simulink model "DREM"  (R2022a)
settings: Solver=FixedStepAuto  StartTime=0.0  StopTime=50.0  FixedStep=0.001  RelTol=1e-6
libraries: cstblocks x3
settings Model: Creator=loryb  LastModifiedBy=loryb

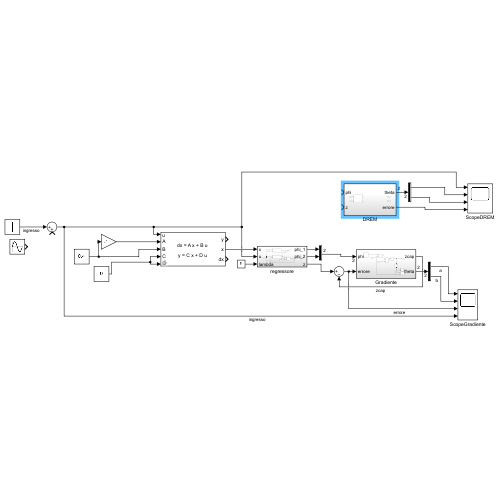
[thumbnail: Simulink's stored preview of the top-level diagram]
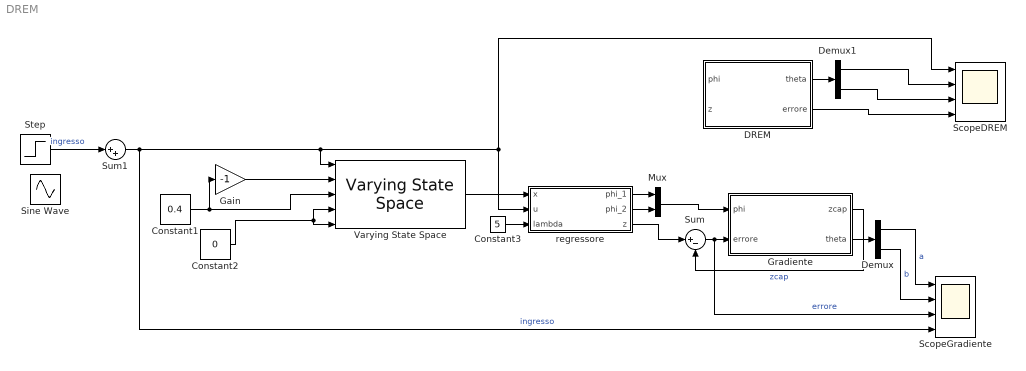
== system DREM ==
  Constant1 : Constant  Value=0.4
  Constant2 : Constant  Value=0
  Constant3 : Constant  Value=5
  DREM : Subsystem
  Demux : Demux  Outputs=2
  Demux1 : Demux  Outputs=2
  Gain : Gain  Gain=-1
  Gradiente : Subsystem
  Mux : Mux  Inputs=2
  ScopeDREM : Scope  NumInputPorts=4
  ScopeGradiente : Scope  NumInputPorts=4
  Sine Wave : Sin  Amplitude=10  Frequency=5/2  SampleTime=0
  Step : Step  Time=3  After=10  SampleTime=0
  Sum : Sum  Inputs=|+-
  Sum1 : Sum  Inputs=|++
  Varying State Space : cstblocks/Linear Parameter Varying/Varying State Space  x0=0  xNames=''  OutputX=on  OutputDX=on
  regressore : Subsystem
  wires:
  Gain/1 -> Varying State Space/2
  Constant1/1 -> Gain/1, Varying State Space/3
  Constant2/1 -> Varying State Space/4, Varying State Space/5
  Varying State Space/2 -> regressore/1(x)
  Constant3/1 -> regressore/3(lambda)
  Sum/1 -> ScopeGradiente/3, Gradiente/2(errore)  "errore"
  Gradiente/1(zcap) -> Sum/2  "zcap"
  regressore/3(z) -> Sum/1
  Sum1/1 -> Varying State Space/1, ScopeDREM/1, regressore/2(u), ScopeGradiente/4  "ingresso"
  Demux/2 -> ScopeGradiente/2  "b"
  Demux/1 -> ScopeGradiente/1  "a"
  regressore/2(phi_2) -> Mux/2
  regressore/1(phi_1) -> Mux/1
  Mux/1 -> Gradiente/1(phi)
  Gradiente/2(theta) -> Demux/1
  Step/1 -> Sum1/1  "ingresso"
  DREM/2(errore) -> ScopeDREM/4
  DREM/1(theta) -> Demux1/1
  Demux1/1 -> ScopeDREM/2
  Demux1/2 -> ScopeDREM/3

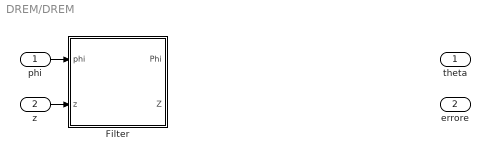
== system DREM/DREM ==
  phi : Inport
  z : Inport  Port=2
  Filter : Subsystem
  theta : Outport
  errore : Outport  Port=2
  wires:
  z/1 -> Filter/2(z)
  phi/1 -> Filter/1(phi)

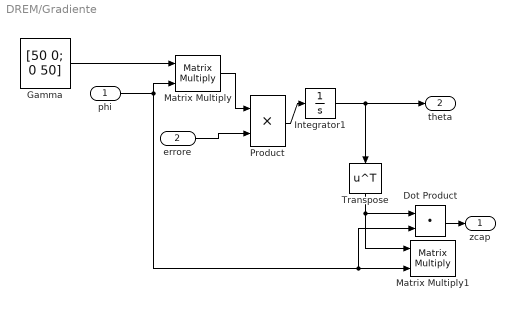
== system DREM/Gradiente ==
  phi : Inport
  errore : Inport  Port=2
  Dot Product : DotProduct  OutDataTypeStr=Inherit: Inherit via internal rule
  Gamma : Constant  Value=[50 0; 0 50]  VectorParams1D=off
  Integrator1 : Integrator
  Matrix Multiply : Product  Multiplication=Matrix(*)
  Matrix Multiply1 : Product  Multiplication=Matrix(*)
  Product : Product
  Transpose : Math  Operator=transpose
  zcap : Outport
  theta : Outport  Port=2
  wires:
  Gamma/1 -> Matrix Multiply/1
  phi/1 -> Matrix Multiply/2, Dot Product/2, Matrix Multiply1/2
  Product/1 -> Integrator1/1
  errore/1 -> Product/2
  Matrix Multiply/1 -> Product/1
  Integrator1/1 -> Transpose/1, theta/1
  Transpose/1 -> Matrix Multiply1/1, Dot Product/1
  Dot Product/1 -> zcap/1

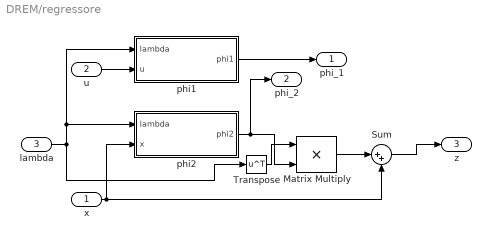
== system DREM/regressore ==
  x : Inport
  u : Inport  Port=2
  lambda : Inport  Port=3
  Matrix Multiply : Product
  Sum : Sum  Inputs=|++
  Transpose : Math  Operator=transpose
  phi1 : Subsystem
  phi2 : Subsystem
  phi_1 : Outport
  phi_2 : Outport  Port=2
  z : Outport  Port=3
  wires:
  x/1 -> Sum/2, phi2/2(x)
  u/1 -> phi1/2(u)
  lambda/1 -> Transpose/1, phi1/1(lambda), phi2/1(lambda)
  phi2/1(phi2) -> Matrix Multiply/2, phi_2/1
  Matrix Multiply/1 -> Sum/1
  Sum/1 -> z/1
  phi1/1(phi1) -> phi_1/1
  Transpose/1 -> Matrix Multiply/1

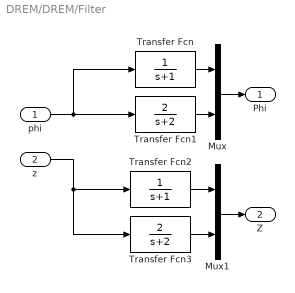
== system DREM/DREM/Filter ==
  phi : Inport
  z : Inport  Port=2
  Mux : Mux  Inputs=2
  Mux1 : Mux  Inputs=2
  Transfer Fcn : TransferFcn  Denominator=[1 1]
  Transfer Fcn1 : TransferFcn  Numerator=[2]  Denominator=[1 2]
  Transfer Fcn2 : TransferFcn  Denominator=[1 1]
  Transfer Fcn3 : TransferFcn  Numerator=[2]  Denominator=[1 2]
  Phi : Outport
  Z : Outport  Port=2
  wires:
  phi/1 -> Transfer Fcn/1, Transfer Fcn1/1
  z/1 -> Transfer Fcn3/1, Transfer Fcn2/1
  Transfer Fcn1/1 -> Mux/2
  Transfer Fcn/1 -> Mux/1
  Transfer Fcn2/1 -> Mux1/1
  Transfer Fcn3/1 -> Mux1/2
  Mux1/1 -> Z/1
  Mux/1 -> Phi/1

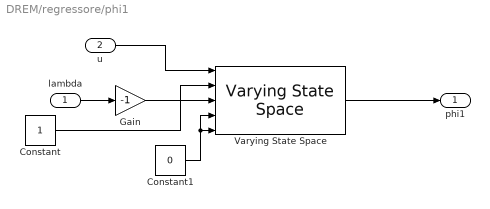
== system DREM/regressore/phi1 ==
  lambda : Inport
  u : Inport  Port=2
  Constant : Constant
  Constant1 : Constant  Value=0
  Gain : Gain  Gain=-1
  Varying State Space : cstblocks/Linear Parameter Varying/Varying State Space  x0=0  xNames=''  OutputX=on  OutputDX=on
  phi1 : Outport
  wires:
  lambda/1 -> Gain/1
  u/1 -> Varying State Space/1
  Gain/1 -> Varying State Space/2
  Constant/1 -> Varying State Space/3
  Varying State Space/2 -> phi1/1
  Constant1/1 -> Varying State Space/5, Varying State Space/4

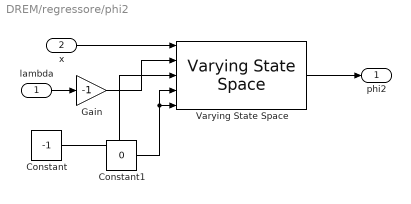
== system DREM/regressore/phi2 ==
  lambda : Inport
  x : Inport  Port=2
  Constant : Constant  Value=-1
  Constant1 : Constant  Value=0
  Gain : Gain  Gain=-1
  Varying State Space : cstblocks/Linear Parameter Varying/Varying State Space  x0=0  xNames=''  OutputX=on  OutputDX=on
  phi2 : Outport
  wires:
  lambda/1 -> Gain/1
  x/1 -> Varying State Space/1
  Gain/1 -> Varying State Space/2
  Constant/1 -> Varying State Space/3
  Varying State Space/2 -> phi2/1
  Constant1/1 -> Varying State Space/5, Varying State Space/4
